simulink library "eulAng2RotMat_ul"  (R2018b)
settings: Solver=VariableStepAuto  StartTime=0.0  StopTime=10.0  RelTol=1e-3
libraries: sharedutil x3
settings Model: Creator=mcobb  LastModifiedBy=mcobb

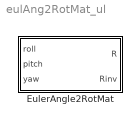
== system eulAng2RotMat_ul ==
  EulerAngle2RotMat : Subsystem

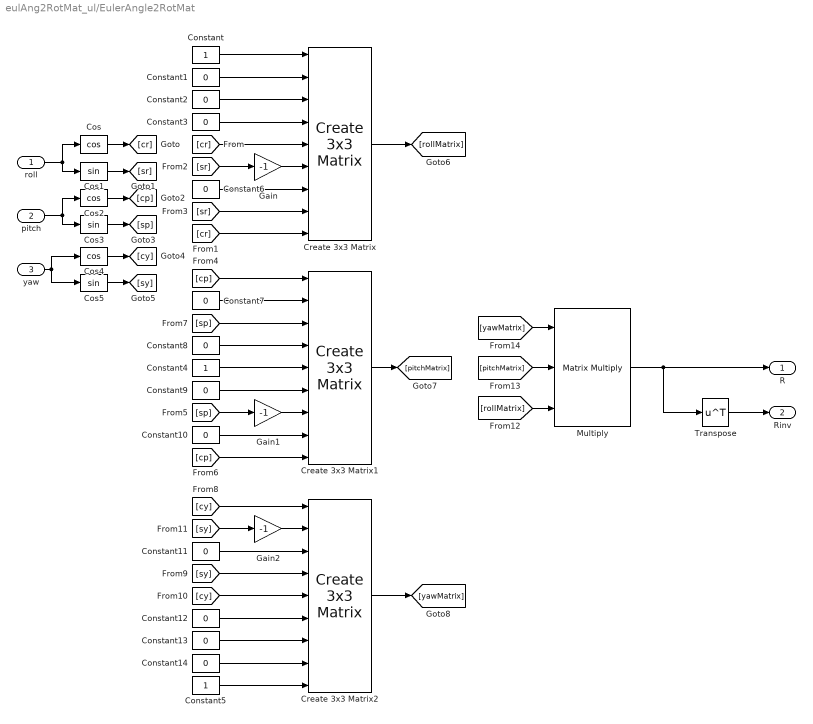
== system eulAng2RotMat_ul/EulerAngle2RotMat ==
  roll : Inport
  pitch : Inport  Port=2
  yaw : Inport  Port=3
  Constant : Constant
  Constant{1..3,6..14} (12 alike) : Constant  Value=0
  Constant4 : Constant
  Constant5 : Constant
  Cos : Trigonometry  Operator=cos
  Cos1 : Trigonometry
  Cos2 : Trigonometry  Operator=cos
  Cos3 : Trigonometry
  Cos4 : Trigonometry  Operator=cos
  Cos5 : Trigonometry
  Create 3x3 Matrix : sharedutil/Create 3x3 Matrix  aMode=aMode
  Create 3x3 Matrix1 : sharedutil/Create 3x3 Matrix  aMode=aMode
  Create 3x3 Matrix2 : sharedutil/Create 3x3 Matrix  aMode=aMode
  Gain : Gain  Gain=-1
  Gain1 : Gain  Gain=-1
  Gain2 : Gain  Gain=-1
  Multiply : Product  Inputs=3  Multiplication=Matrix(*)
  Transpose : Math  Operator=transpose  SaturateOnIntegerOverflow=on
  R : Outport
  Rinv : Outport  Port=2
  wires:
  roll/1 -> Cos/1, Cos1/1
  Cos/1 -> [cr]
  Cos1/1 -> [sr]
  pitch/1 -> Cos3/1, Cos2/1
  yaw/1 -> Cos4/1, Cos5/1
  Cos2/1 -> [cp]
  Cos3/1 -> [sp]
  Cos4/1 -> [cy]
  Cos5/1 -> [sy]
  Constant/1 -> Create 3x3 Matrix/1
  Constant1/1 -> Create 3x3 Matrix/2
  [cr] -> Create 3x3 Matrix/5
  [cr] -> Create 3x3 Matrix/9
  [sr] -> Gain/1
  [sr] -> Create 3x3 Matrix/8
  Constant3/1 -> Create 3x3 Matrix/4
  Constant2/1 -> Create 3x3 Matrix/3
  Constant6/1 -> Create 3x3 Matrix/7
  Gain/1 -> Create 3x3 Matrix/6
  Create 3x3 Matrix/1 -> [rollMatrix]
  Constant4/1 -> Create 3x3 Matrix1/5
  Constant5/1 -> Create 3x3 Matrix2/9
  Constant7/1 -> Create 3x3 Matrix1/2
  Constant8/1 -> Create 3x3 Matrix1/4
  Constant9/1 -> Create 3x3 Matrix1/6
  Constant10/1 -> Create 3x3 Matrix1/8
  Constant11/1 -> Create 3x3 Matrix2/3
  Constant12/1 -> Create 3x3 Matrix2/6
  Constant13/1 -> Create 3x3 Matrix2/7
  Constant14/1 -> Create 3x3 Matrix2/8
  [cp] -> Create 3x3 Matrix1/1
  [cp] -> Create 3x3 Matrix1/9
  [sp] -> Gain1/1
  [sp] -> Create 3x3 Matrix1/3
  Gain1/1 -> Create 3x3 Matrix1/7
  [cy] -> Create 3x3 Matrix2/1
  [cy] -> Create 3x3 Matrix2/5
  [sy] -> Create 3x3 Matrix2/4
  [sy] -> Gain2/1
  Gain2/1 -> Create 3x3 Matrix2/2
  Create 3x3 Matrix1/1 -> [pitchMatrix]
  Create 3x3 Matrix2/1 -> [yawMatrix]
  [rollMatrix] -> Multiply/3
  [pitchMatrix] -> Multiply/2
  [yawMatrix] -> Multiply/1
  Multiply/1 -> Transpose/1, R/1
  Transpose/1 -> Rinv/1
